simulink model "actuator"  (R2022b)
settings: Solver=FixedStepAuto  StartTime=0.0  StopTime=t_max  FixedStep=timestep  RelTol=1e-3
values from neighbouring files (symbols this model uses):
  A = [ 0 1  0 ... (first row only)    [script.m]
  a1 = -(Ra/La) - (Bt/Ja)    (= -112.440298507)    [script.m]
  a2 = -(Ra*Bt+Ce*Ca)/(La*Ja)    (= -188.339552239)    [script.m]
  B = [0; 0; fwu]    [script.m]
  C = ones(q,n)    [script.m]
  D = zeros(q,p)    [script.m]
  K = sym2poly(K(1))    [script.m]
  La = 0.067    [script.m]
  Ra = 7.5    [script.m]
  step_v = 1    [script.m]
  timestep = t_max/1e6    (= 4e-05)    [script.m]
libraries: simulink x1
settings Model: Creator=mluser  LastModifiedBy=mluser

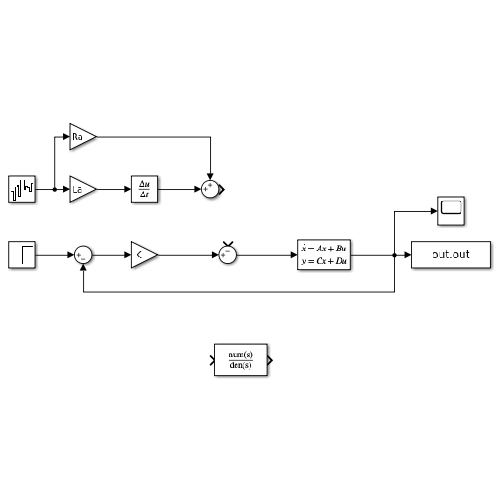
[thumbnail: Simulink's stored preview of the top-level diagram]
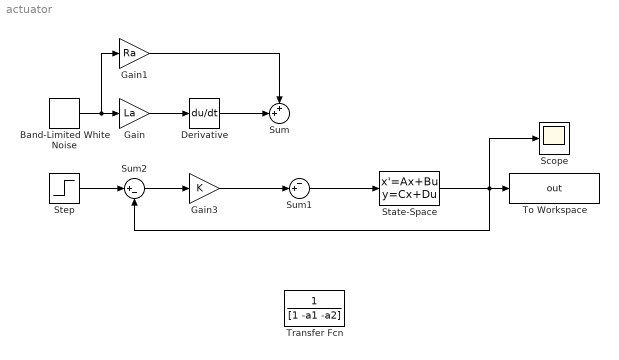
== system actuator ==
  Band-Limited White Noise : simulink/Sources/Band-Limited White Noise  Cov=step_v  Ts=timestep  seed=[23341]
  Derivative : Derivative
  Gain : Gain  Gain=La
  Gain1 : Gain  Gain=Ra
  Gain3 : Gain  Gain=K
  Scope : Scope
  State-Space : StateSpace  A=A  B=B  C=C  D=D  InitialCondition=0
  Step : Step  Time=0  After=step_v  SampleTime=0
  Sum : Sum  Inputs=++|
  Sum1 : Sum  Inputs=-+|
  Sum2 : Sum  Inputs=|+-
  To Workspace : ToWorkspace  VariableName=out  SampleTime=-1
  Transfer Fcn : TransferFcn  Numerator=1  Denominator=[1 -a1 -a2]
  wires:
  Derivative/1 -> Sum/2
  Gain/1 -> Derivative/1
  Band-Limited White Noise/1 -> Gain1/1, Gain/1
  Gain1/1 -> Sum/1
  Gain3/1 -> Sum1/2
  State-Space/1 -> Sum2/2, Scope/1, To Workspace/1
  Sum2/1 -> Gain3/1
  Step/1 -> Sum2/1
  Sum1/1 -> State-Space/1
